simulink model "RPS_HW_2025"  (R2024b)
settings: Solver=FixedStepAuto  StartTime=0.0  StopTime=inf  RelTol=1e-3
libraries: microbitledlib x5, microbitaccellib x2
settings Model: SimulationMode=external  ExtModeTrigDuration=5  Creator=avizinho  LastModifiedBy=ahenshaw
settings SolverCC: AlgebraicLoopSolver=TrustRegion
settings DataIOCC: ReturnWorkspaceOutputs=off
settings OptimizationCC: EnhancedBackFolding=on  PassReuseOutputArgsThreshold=0  MaxStackSize=64  OptimizeBlockOrder=speed  DifferentSizesBufferReuse=on  OptimizationCustomize=off
settings DebuggingCC: ParameterTunabilityLossMsg=error  UnconnectedInputMsg=warning  UnconnectedOutputMsg=warning  UnconnectedLineMsg=warning  ArithmeticOperatorsInVariantConditions=warning
settings HardwareCC: ProdBitPerPointer=32  ProdBitPerSizeT=32  ProdBitPerPtrDiffT=32  ProdLargestAtomicInteger=Long  ProdLargestAtomicFloat=Double  ProdWordSize=32  ProdHWDeviceType=ARM Compatible->ARM Cortex
settings ModelReferenceCC: EnableRefExpFcnMdlSchedulingChecks=on
settings SFSimCC: MATLABDynamicMemAlloc=off  CustomCodeUndefinedFunction=UseInterfaceOnly
settings RTWCC: Description=Embedded Coder  SystemTargetFile=ert.tlc  HardwareBoard=BBC micro:bit V2  TemplateMakefile=ert_default_tmf  Toolchain=GNU Tools for ARM Embedded Processors  GPUComputeCapability=3.5
settings CodeAppCC: ForceParamTrailComments=on  OperatorAnnotations=on
settings ERTTargetCC: ERTCustomFileBanners=off  SupportContinuousTime=on  SupportNonInlinedSFcns=on  RemoveResetFunc=off  ModelStepFunctionPrototypeControlCompliant=off  ExtModeTransport=3  ExtModeStaticAlloc=on  ExtModeMexFile=ext_xcp  ExtModeIntrfLevel=Level2 - Open  InlinedParameterPlacement=Hierarchical  DynamicArrayContainerType=coder::array

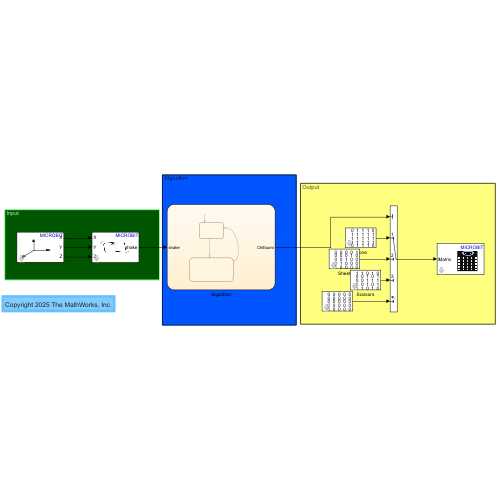
[thumbnail: Simulink's stored preview of the top-level diagram]
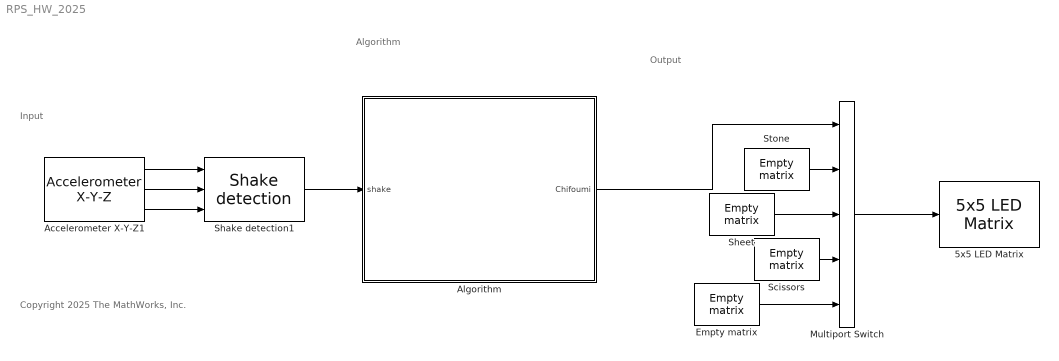
== system RPS_HW_2025 ==
  note: Output
  note: Algorithm
  note: Input
  note: Copyright 2025 The MathWorks, Inc.
  5x5 LED Matrix : microbitledlib/5x5 LED Matrix  LED_mat=[0 1 1 1 0;1 0 1 0 1;1 1 0 1 1; 1 0 1 0 1;0 1 1 1 0]
  Accelerometer X-Y-Z1 : microbitaccellib/Accelerometer X-Y-Z  ODR=800Hz  Accelfullrange=-2g to +2g  SampleTime=0.1
  Algorithm : Stateflow chart  TreatAsAtomicUnit=on
  Empty matrix : microbitledlib/LED Images/Empty matrix  L00=off  L01=off  L02=off  L03=off  L04=off  L10=off  L11=off  L12=off  L13=off  L14=off  L20=off  L21=off  L22=off  L23=off  L24=off  L30=off  L31=off  L32=off  L33=off  L34=off  L40=off  L41=off  L42=off  L43=off  L44=off
  Multiport Switch : MultiPortSwitch  Inputs=4  SaturateOnIntegerOverflow=off  InputSameDT=off
  Scissors : microbitledlib/LED Images/Empty matrix  L00=on  L01=on  L02=off  L03=on  L04=off  L10=off  L11=off  L12=on  L13=off  L14=on  L20=off  L21=off  L22=on  L23=on  L24=on  L30=off  L31=off  L32=on  L33=off  L34=on  L40=on  L41=on  L42=off  L43=on  L44=off
  Shake detection1 : microbitaccellib/Shake detection  sen=3
  Sheet : microbitledlib/LED Images/Empty matrix  L00=off  L01=off  L02=off  L03=off  L04=on  L10=off  L11=off  L12=off  L13=on  L14=off  L20=off  L21=off  L22=on  L23=off  L24=off  L30=off  L31=on  L32=off  L33=off  L34=off  L40=on  L41=off  L42=off  L43=off  L44=off
  Stone : microbitledlib/LED Images/Empty matrix  L00=off  L01=on  L02=on  L03=on  L04=off  L10=on  L11=on  L12=on  L13=on  L14=on  L20=on  L21=on  L22=on  L23=on  L24=on  L30=on  L31=on  L32=on  L33=on  L34=on  L40=off  L41=on  L42=on  L43=on  L44=off
  wires:
  Algorithm/1(Chifoumi) -> Multiport Switch/1
  Shake detection1/1 -> Algorithm/1(shake)
  Accelerometer X-Y-Z1/1 -> Shake detection1/1
  Accelerometer X-Y-Z1/2 -> Shake detection1/2
  Accelerometer X-Y-Z1/3 -> Shake detection1/3
  Multiport Switch/1 -> 5x5 LED Matrix/1
  Stone/1 -> Multiport Switch/2
  Sheet/1 -> Multiport Switch/3
  Scissors/1 -> Multiport Switch/4
  Empty matrix/1 -> Multiport Switch/5

== stateflow chart RPS_HW_2025/Algorithm ==
  state Start
    Chifoumi=0;
  state Play
    entry: Chifoumi=randi(3);
  (default) -> Start
  Play -> Start : after(3,sec)
  Start -> Play : [shake==1]
  data: Chifoumi output; shake input
